simulink model "Ex1_Comparacion_con_SVC_Simulink"  (R2019a)
settings: Solver=VariableStepAuto  StartTime=0.0  StopTime=1  RelTol=1e-3
libraries: powerlib x53, powerlib_meascontrol x10, factslib x1
settings Model: Creator=USUARIO  LastModifiedBy=USUARIO

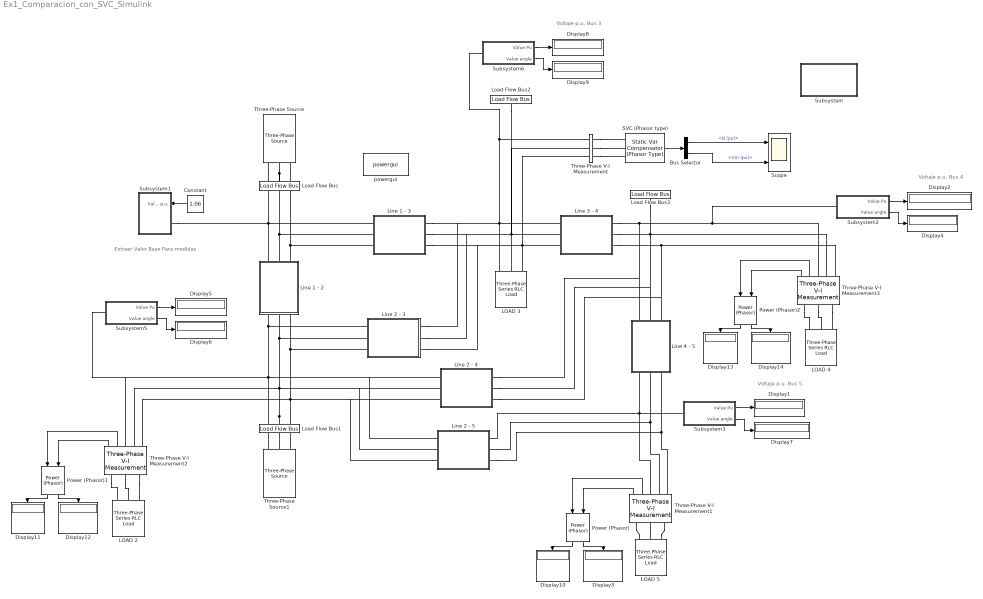
== system Ex1_Comparacion_con_SVC_Simulink ==
  note: Voltaje p.u. Bus 4
  note: Extraer Valor Base Para medidas
  note: Voltaje p.u. Bus 5
  note: Voltaje p.u. Bus 3
  Bus Selector : BusSelector  OutputSignals=Control.B (pu),Control.Vm (pu)
  Constant : Constant  Value=1.06
  Display{1..14} (14 alike) : Display
  LOAD 2 : powerlib/Elements/Three-Phase Series RLC Load  LConnTagsString=A|B|C  Configuration=Y (grounded)  NominalVoltage=(10000)*1  Vabc=[1e3 1e3 1e3]  Vabcp=[1e3 1e3 1e3]  NominalFrequency=60  UnbalancedPower=off  ActivePower=20e6  InductivePower=10e6  CapacitivePower=0  Pabc=[10e3 9e3 11e3]  QLabc=[100 90 110]  QCabc=[100 90 110]  Pabcp=[10e3 9e3 11e3]  QLabcp=[100 90 110]  QCabcp=[100 90 110]  Measurements=None  LoadType=constant PQ
      settings: SourceProductName=Simscape Electrical
  LOAD 3 : powerlib/Elements/Three-Phase Series RLC Load  LConnTagsString=A|B|C  Configuration=Y (grounded)  NominalVoltage=(10000)  Vabc=[1e3 1e3 1e3]  Vabcp=[1e3 1e3 1e3]  NominalFrequency=60  UnbalancedPower=off  ActivePower=45e6  InductivePower=15e6  CapacitivePower=0  Pabc=[10e3 9e3 11e3]  QLabc=[100 90 110]  QCabc=[100 90 110]  Pabcp=[10e3 9e3 11e3]  QLabcp=[100 90 110]  QCabcp=[100 90 110]  Measurements=None  LoadType=constant PQ
      settings: SourceProductName=Simscape Electrical
  LOAD 4 : powerlib/Elements/Three-Phase Series RLC Load  LConnTagsString=A|B|C  Configuration=Y (grounded)  NominalVoltage=(10000)*0.9943897  Vabc=[1e3 1e3 1e3]  Vabcp=[1e3 1e3 1e3]  NominalFrequency=60  UnbalancedPower=off  ActivePower=40e6  InductivePower=5e6  CapacitivePower=0  Pabc=[10e3 9e3 11e3]  QLabc=[100 90 110]  QCabc=[100 90 110]  Pabcp=[10e3 9e3 11e3]  QLabcp=[100 90 110]  QCabcp=[100 90 110]  Measurements=None  LoadType=constant PQ
      settings: SourceProductName=Simscape Electrical
  LOAD 5 : powerlib/Elements/Three-Phase Series RLC Load  LConnTagsString=A|B|C  Configuration=Y (grounded)  NominalVoltage=(10000)*0.9753  Vabc=[1e3 1e3 1e3]  Vabcp=[1e3 1e3 1e3]  NominalFrequency=60  UnbalancedPower=off  ActivePower=60e6  InductivePower=10e6  CapacitivePower=0  Pabc=[10e3 9e3 11e3]  QLabc=[100 90 110]  QCabc=[100 90 110]  Pabcp=[10e3 9e3 11e3]  QLabcp=[100 90 110]  QCabcp=[100 90 110]  Measurements=None  LoadType=constant PQ
      settings: SourceProductName=Simscape Electrical
  "Line 1 - 2 " : Subsystem  mask{F=60, R=0.02, XL=0.06, B=0.03}
      mask prompts: F "Frequency"; R "Resistance"; XL "Reactance"; B "Susceptance"
      mask Display: disp('Line')
  Line 1 - 3 : Subsystem  mask{F=60, R=0.08, XL=0.24, B=0.025}
      mask prompts: F "Frequency"; R "Resistance"; XL "Reactance"; B "Susceptance"
      mask Display: disp('Line')
  Line 2 - 3 : Subsystem  mask{F=60, R=0.06, XL=0.18, B=0.02}
      mask prompts: F "Frequency"; R "Resistance"; XL "Reactance"; B "Susceptance"
      mask Display: disp('Line')
  Line 2 - 4 : Subsystem  mask{F=60, R=0.06, XL=0.18, B=0.02}
      mask prompts: F "Frequency"; R "Resistance"; XL "Reactance"; B "Susceptance"
      mask Display: disp('Line')
  Line 2 - 5 : Subsystem  mask{F=60, R=0.04, XL=0.12, B=0.015}
      mask prompts: F "Frequency"; R "Resistance"; XL "Reactance"; B "Susceptance"
      mask Display: disp('Line')
  Line 3 - 4 : Subsystem  mask{F=60, R=0.01, XL=0.03, B=0.01}
      mask prompts: F "Frequency"; R "Resistance"; XL "Reactance"; B "Susceptance"
      mask Display: disp('Line')
  Line 4 - 5 : Subsystem  mask{F=60, R=0.08, XL=0.24, B=0.025}
      mask prompts: F "Frequency"; R "Resistance"; XL "Reactance"; B "Susceptance"
      mask Display: disp('Line')
  Load Flow Bus : powerlib/Measurements/Load Flow Bus  LConnTagsString=a  Phases=single  Connectors=on one side  ID=BUS_1  Vbase=10e3  Vref=1.06  Vangle=0  VLF=1.06  VLFb=1  VLFc=1  angleLF=0  angleLFb=0  angleLFc=0
      settings: SourceProductName=Simscape Electrical
  Load Flow Bus1 : powerlib/Measurements/Load Flow Bus  LConnTagsString=a  Phases=single  Connectors=on one side  ID=BUS_2  Vbase=10e3  Vref=1  Vangle=0  VLF=1  VLFb=1  VLFc=1  angleLF=-2.061  angleLFb=0  angleLFc=0
      settings: SourceProductName=Simscape Electrical
  Load Flow Bus2 : powerlib/Measurements/Load Flow Bus  LConnTagsString=a  Phases=single  Connectors=on one side  ID=BUS_3  Vbase=10e3  Vref=1  Vangle=0  VLF=0.9872  VLFb=1  VLFc=1  angleLF=-4.637  angleLFb=0  angleLFc=0
      settings: SourceProductName=Simscape Electrical
  Load Flow Bus3 : powerlib/Measurements/Load Flow Bus  LConnTagsString=a  Phases=single  Connectors=on one side  ID=BUS_4  Vbase=10e3  Vref=1  Vangle=0  VLF=0.9841  VLFb=1  VLFc=1  angleLF=-4.957  angleLFb=0  angleLFc=0
      settings: SourceProductName=Simscape Electrical
  Power (Phasor) : powerlib_meascontrol/Measurements/Power (Phasor)
      settings: SourceProductName=Simscape Electrical  SourceProductBaseCode=PS
  Power (Phasor)1 : powerlib_meascontrol/Measurements/Power (Phasor)
      settings: SourceProductName=Simscape Electrical  SourceProductBaseCode=PS
  Power (Phasor)2 : powerlib_meascontrol/Measurements/Power (Phasor)
      settings: SourceProductName=Simscape Electrical  SourceProductBaseCode=PS
  SVC (Phasor type) : factslib/Power-Electronics Based FACTS/Static Var Compensator (Phasor Type)  Seq1_Only=on  SystemNominal="[10e3  60]"  Pbase=200e6  Qnom="[200e6  -100e6]"  Td=4e-3  mode=Voltage regulation  Vref=1.0  ExternalVref=off  Xs=0  Kp_Ki=[0 300]  Bref=0.0
      settings: SourceProductName=Simscape Electrical  SourceProductBaseCode=PS
  Scope : Scope  NumInputPorts=2
  Subsystem : Subsystem
      mask Display: disp('Signal Processing')
  Subsystem1 : Subsystem
  Subsystem2 : Subsystem
  Subsystem3 : Subsystem
  Subsystem5 : Subsystem
  Subsystem6 : Subsystem
  Three-Phase V-I Measurement : powerlib/Measurements/Three-Phase V-I Measurement  VoltageMeasurement=phase-to-ground  SetLabelV=on  LabelV=Vabc  Vpu=on  VpuLL=off  CurrentMeasurement=yes  SetLabelI=on  LabelI=Iabc  Ipu=on  Pbase=100e6  Vbase=500e3  OutputType=Complex  PhasorSimulation=on  PSBequivalent=0
      settings: SourceProductName=Simscape Electrical
  Three-Phase V-I Measurement1 : powerlib/Measurements/Three-Phase V-I Measurement  VoltageMeasurement=phase-to-ground  SetLabelV=off  LabelV=Vabc  Vpu=off  VpuLL=off  CurrentMeasurement=yes  SetLabelI=off  LabelI=Iabc  Ipu=off  Pbase=100e6  Vbase=500e3  OutputType=Complex  PhasorSimulation=on  PSBequivalent=0
      settings: SourceProductName=Simscape Electrical
  Three-Phase V-I Measurement2 : powerlib/Measurements/Three-Phase V-I Measurement  VoltageMeasurement=phase-to-ground  SetLabelV=off  LabelV=Vabc  Vpu=off  VpuLL=off  CurrentMeasurement=yes  SetLabelI=off  LabelI=Iabc  Ipu=off  Pbase=100e6  Vbase=500e3  OutputType=Complex  PhasorSimulation=on  PSBequivalent=0
      settings: SourceProductName=Simscape Electrical
  Three-Phase V-I Measurement3 : powerlib/Measurements/Three-Phase V-I Measurement  VoltageMeasurement=phase-to-ground  SetLabelV=off  LabelV=Vabc  Vpu=off  VpuLL=off  CurrentMeasurement=yes  SetLabelI=off  LabelI=Iabc  Ipu=off  Pbase=100e6  Vbase=500e3  OutputType=Complex  PhasorSimulation=on  PSBequivalent=0
      settings: SourceProductName=Simscape Electrical
  Three-Phase Source : powerlib/Electrical Sources/Three-Phase Source  InternalConnection=Yg  VoltagePhases=off  Voltage=(10000)*1.06  PhaseAngle=0  Voltage_phases=[25e3 25e3 25e3]/sqrt(3)  PhaseAngles_phases=[0 -120 +120]  Frequency=60  NonIdealSource=off  SpecifyImpedance=off  Resistance=1e-5  Inductance=0  ShortCircuitLevel=100e6  BaseVoltage=10e3  XRratio=7  BusType=swing  Pref=10e3  Qref=0  Prefabc=[10e3, 10e3, 10e3]  Qrefabc=[0, 0, 0]  Qmin=-inf  Qmax=inf
      settings: SourceProductName=Simscape Electrical
  Three-Phase Source1 : powerlib/Electrical Sources/Three-Phase Source  InternalConnection=Yg  VoltagePhases=off  Voltage=(10000)*1  PhaseAngle=-2.053  Voltage_phases=[25e3 25e3 25e3]/sqrt(3)  PhaseAngles_phases=[0 -120 +120]  Frequency=60  NonIdealSource=off  SpecifyImpedance=off  Resistance=0.8929  Inductance=16.58e-3  ShortCircuitLevel=100e6  BaseVoltage=25e3  XRratio=7  BusType=PV  Pref=40e6  Qref=0  Prefabc=[10e3, 10e3, 10e3]  Qrefabc=[0, 0, 0]  Qmin=-inf  Qmax=inf
      settings: SourceProductName=Simscape Electrical
  powergui : powerlib/powergui  Priority=1  SimulationMode=Phasor  SampleTime=50e-6  frequency=60  Iterations=50  frequencyindice=60  Pbase=100e6  ErrMax=1e-12  UnitsV=kV  UnitsW=MW  buscounter=0  FunctionMessages=off  echomessages=off  EnableUseOfTLC=off  CurrentSourceSwitches=off  DisableSnubberDevices=off  DisableRonSwitches=off  DisableVfSwitches=off  DisplayEquations=off  AutomaticDiscreteSolvers=off  SolverType=Tustin/Backward Euler (TBE)  Interpol=off  ExternalGateDelay=off  methode=off  Ts=100  x0status=blocks  SPID=on  SwTol=0  HookPort=off  NonlinearTolerance=0  nMaxIteration=15  ContinueOnMaxIteration=off  RestoreLinks=warning  ResistiveCurrentMeasurement=off  Frange=[0:2:500]  Ylog=off  Xlog=on  ShowGrid=off  save=off  variable=ZData  structure=0  ZoomFFT=off  StartTime=0.0  cycles=1  DisplayStyle=1  fundamental=60  FreqAxis=off  MaxFrequency=1000  frequencyindicesteady=1  RmsSteady=1  display=off
      settings: SourceProductName=Simscape Electrical
  wires:
  SVC (Phasor type)/1 -> Bus Selector/1
  Bus Selector/2 -> Scope/2  "<Vm (pu)>"
  Bus Selector/1 -> Scope/1  "<B (pu)>"
  Constant/1 -> Subsystem1/1(Value p.u.)
  Subsystem2/2(Value angle) -> Display4/1
  Subsystem5/2(Value angle) -> Display6/1
  Subsystem5/1("Value Pu ") -> Display5/1
  Subsystem3/2(Value angle) -> Display7/1
  Subsystem3/1("Value Pu ") -> Display1/1
  Subsystem6/1("Value Pu ") -> Display8/1
  Subsystem6/2(Value angle) -> Display9/1
  Subsystem2/1("Value Pu ") -> Display2/1
  Power (Phasor)/2 -> Display10/1
  Power (Phasor)/1 -> Display3/1
  Three-Phase V-I Measurement1/1 -> Power (Phasor)/1
  Three-Phase V-I Measurement1/2 -> Power (Phasor)/2
  Three-Phase V-I Measurement2/2 -> Power (Phasor)1/2
  Power (Phasor)1/1 -> Display12/1
  Power (Phasor)1/2 -> Display11/1
  Three-Phase V-I Measurement2/1 -> Power (Phasor)1/1
  Three-Phase V-I Measurement3/2 -> Power (Phasor)2/2
  Power (Phasor)2/1 -> Display14/1
  Power (Phasor)2/2 -> Display13/1
  Three-Phase V-I Measurement3/1 -> Power (Phasor)2/1
  connections:
  Three-Phase Source1/RConn1 -- Three-Phase V-I Measurement2/RConn1 -- Subsystem5/LConn1 -- Line 2 - 5/LConn1 -- Line 2 - 4/LConn1 -- "Line 1 - 2 "/RConn1 -- Line 2 - 3/LConn1
  Three-Phase Source1/RConn2 -- Load Flow Bus1/LConn1 -- Three-Phase V-I Measurement2/RConn2 -- Line 2 - 4/LConn2 -- Line 2 - 5/LConn2 -- "Line 1 - 2 "/RConn2 -- Line 2 - 3/LConn2
  Three-Phase Source1/RConn3 -- Three-Phase V-I Measurement2/RConn3 -- "Line 1 - 2 "/RConn3 -- Line 2 - 3/LConn3 -- Line 2 - 4/LConn3 -- Line 2 - 5/LConn3
  Load Flow Bus/LConn1 -- Line 1 - 3/LConn2 -- "Line 1 - 2 "/LConn2 -- Three-Phase Source/RConn2
  Line 1 - 3/LConn3 -- Three-Phase Source/RConn3 -- "Line 1 - 2 "/LConn3
  LOAD 3/LConn1 -- Subsystem6/LConn1 -- Three-Phase V-I Measurement/LConn1 -- Line 3 - 4/LConn1 -- Line 2 - 3/RConn1 -- Line 1 - 3/RConn1
  LOAD 3/LConn2 -- Load Flow Bus2/LConn1 -- Three-Phase V-I Measurement/LConn2 -- Line 3 - 4/LConn2 -- Line 2 - 3/RConn2 -- Line 1 - 3/RConn2
  LOAD 3/LConn3 -- Three-Phase V-I Measurement/LConn3 -- Line 3 - 4/LConn3 -- Line 2 - 3/RConn3 -- Line 1 - 3/RConn3
  Line 3 - 4/RConn1 -- Line 4 - 5/LConn1 -- Line 2 - 4/RConn1 -- Three-Phase V-I Measurement3/RConn1 -- Subsystem2/LConn1
  Line 3 - 4/RConn2 -- Three-Phase V-I Measurement3/RConn2 -- Load Flow Bus3/LConn1 -- Line 4 - 5/LConn2 -- Line 2 - 4/RConn2
  Line 3 - 4/RConn3 -- Three-Phase V-I Measurement3/RConn3 -- Line 2 - 4/RConn3 -- Line 4 - 5/LConn3
  Line 2 - 5/RConn1 -- Three-Phase V-I Measurement1/RConn1 -- Subsystem3/LConn1 -- Line 4 - 5/RConn1
  Line 2 - 5/RConn2 -- Three-Phase V-I Measurement1/RConn2 -- Line 4 - 5/RConn2
  Line 2 - 5/RConn3 -- Three-Phase V-I Measurement1/RConn3 -- Line 4 - 5/RConn3
  Three-Phase V-I Measurement/RConn2 -- SVC (Phasor type)/LConn2
  Three-Phase V-I Measurement/RConn3 -- SVC (Phasor type)/LConn3
  Three-Phase V-I Measurement/RConn1 -- SVC (Phasor type)/LConn1
  Line 1 - 3/LConn1 -- Subsystem1/LConn1 -- Three-Phase Source/RConn1 -- "Line 1 - 2 "/LConn1
  Three-Phase V-I Measurement1/LConn1 -- LOAD 5/LConn1
  Three-Phase V-I Measurement1/LConn2 -- LOAD 5/LConn2
  Three-Phase V-I Measurement1/LConn3 -- LOAD 5/LConn3
  Three-Phase V-I Measurement2/LConn3 -- LOAD 2/LConn3
  Three-Phase V-I Measurement2/LConn1 -- LOAD 2/LConn1
  Three-Phase V-I Measurement2/LConn2 -- LOAD 2/LConn2
  Three-Phase V-I Measurement3/LConn1 -- LOAD 4/LConn1
  Three-Phase V-I Measurement3/LConn2 -- LOAD 4/LConn2
  Three-Phase V-I Measurement3/LConn3 -- LOAD 4/LConn3

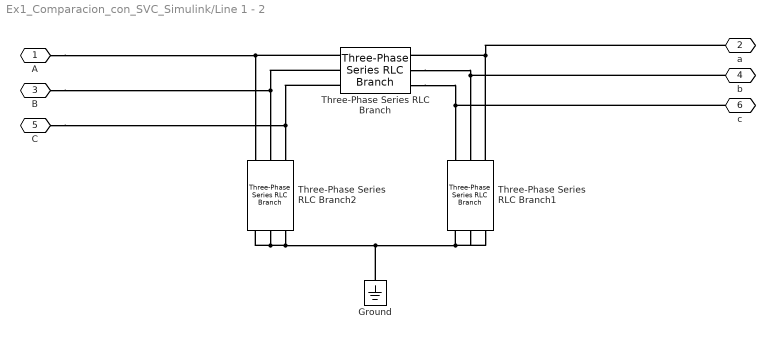
== system Ex1_Comparacion_con_SVC_Simulink/Line 1 - 2  ==
  Ground : powerlib/Elements/Ground  LConnTagsString=a
      settings: SourceProductName=Simscape Electrical
  Three-Phase Series RLC Branch : powerlib/Elements/Three-Phase Series RLC Branch  LConnTagsString=A|B|C  RConnTagsString=A|B|C  BranchType=RL  Resistance=R  Inductance=XL/(2*pi*F)  Capacitance=0  Measurements=None
      settings: SourceProductName=Simscape Electrical
  Three-Phase Series RLC Branch1 : powerlib/Elements/Three-Phase Series RLC Branch  LConnTagsString=A|B|C  RConnTagsString=A|B|C  BranchType=RC  Resistance=1e-5  Inductance=0  Capacitance=B/(2*pi*F)  Measurements=None
      settings: SourceProductName=Simscape Electrical
  Three-Phase Series RLC Branch2 : powerlib/Elements/Three-Phase Series RLC Branch  LConnTagsString=A|B|C  RConnTagsString=A|B|C  BranchType=RC  Resistance=1e-5  Inductance=0  Capacitance=B/(2*pi*F)  Measurements=None
      settings: SourceProductName=Simscape Electrical
  A : PMIOPort  Side=Left
  a : PMIOPort  Port=2  Side=Right
  B : PMIOPort  Port=3  Side=Left
  b : PMIOPort  Port=4  Side=Right
  C : PMIOPort  Port=5  Side=Left
  c : PMIOPort  Port=6  Side=Right
  connections:
  Three-Phase Series RLC Branch/RConn3 -- c/RConn1 -- Three-Phase Series RLC Branch1/LConn1
  Three-Phase Series RLC Branch2/RConn3 -- Ground/LConn1 -- Three-Phase Series RLC Branch1/RConn3 -- Three-Phase Series RLC Branch1/RConn2 -- Three-Phase Series RLC Branch1/RConn1 -- Three-Phase Series RLC Branch2/RConn2 -- Three-Phase Series RLC Branch2/RConn1
  Three-Phase Series RLC Branch/LConn3 -- C/RConn1 -- Three-Phase Series RLC Branch2/LConn3
  Three-Phase Series RLC Branch1/LConn3 -- a/RConn1 -- Three-Phase Series RLC Branch/RConn1
  Three-Phase Series RLC Branch/RConn2 -- b/RConn1 -- Three-Phase Series RLC Branch1/LConn2
  Three-Phase Series RLC Branch/LConn2 -- B/RConn1 -- Three-Phase Series RLC Branch2/LConn2
  Three-Phase Series RLC Branch/LConn1 -- A/RConn1 -- Three-Phase Series RLC Branch2/LConn1

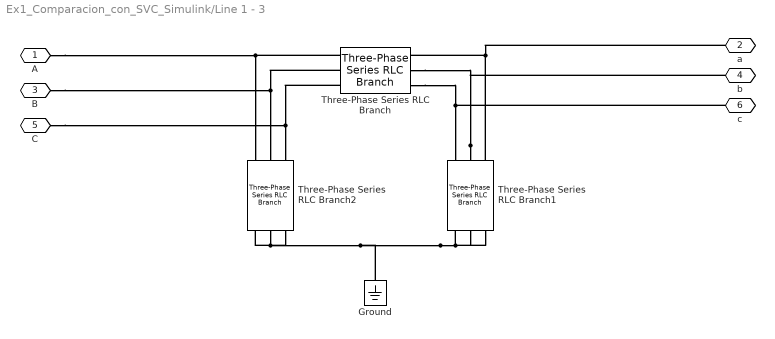
== system Ex1_Comparacion_con_SVC_Simulink/Line 1 - 3 ==
  Ground : powerlib/Elements/Ground  LConnTagsString=a
      settings: SourceProductName=Simscape Electrical
  Three-Phase Series RLC Branch : powerlib/Elements/Three-Phase Series RLC Branch  LConnTagsString=A|B|C  RConnTagsString=A|B|C  BranchType=RL  Resistance=R  Inductance=XL/(2*pi*F)  Capacitance=0  Measurements=None
      settings: SourceProductName=Simscape Electrical
  Three-Phase Series RLC Branch1 : powerlib/Elements/Three-Phase Series RLC Branch  LConnTagsString=A|B|C  RConnTagsString=A|B|C  BranchType=C  Resistance=0  Inductance=0  Capacitance=B/(2*pi*F)  Measurements=None
      settings: SourceProductName=Simscape Electrical
  Three-Phase Series RLC Branch2 : powerlib/Elements/Three-Phase Series RLC Branch  LConnTagsString=A|B|C  RConnTagsString=A|B|C  BranchType=RC  Resistance=1e-5  Inductance=0  Capacitance=B/(2*pi*F)  Measurements=None
      settings: SourceProductName=Simscape Electrical
  A : PMIOPort  Side=Left
  a : PMIOPort  Port=2  Side=Right
  B : PMIOPort  Port=3  Side=Left
  b : PMIOPort  Port=4  Side=Right
  C : PMIOPort  Port=5  Side=Left
  c : PMIOPort  Port=6  Side=Right
  connections:
  Three-Phase Series RLC Branch/RConn3 -- Three-Phase Series RLC Branch1/LConn1 -- c/RConn1
  Three-Phase Series RLC Branch2/RConn2 -- Three-Phase Series RLC Branch2/RConn1 -- Three-Phase Series RLC Branch2/RConn3 -- Three-Phase Series RLC Branch1/RConn3 -- Three-Phase Series RLC Branch1/RConn2 -- Three-Phase Series RLC Branch1/RConn1 -- Ground/LConn1
  Three-Phase Series RLC Branch/LConn3 -- Three-Phase Series RLC Branch2/LConn3 -- C/RConn1
  Three-Phase Series RLC Branch1/LConn3 -- Three-Phase Series RLC Branch/RConn1 -- a/RConn1
  Three-Phase Series RLC Branch1/LConn2 -- Three-Phase Series RLC Branch/RConn2 -- b/RConn1
  Three-Phase Series RLC Branch/LConn2 -- Three-Phase Series RLC Branch2/LConn2 -- B/RConn1
  Three-Phase Series RLC Branch/LConn1 -- Three-Phase Series RLC Branch2/LConn1 -- A/RConn1

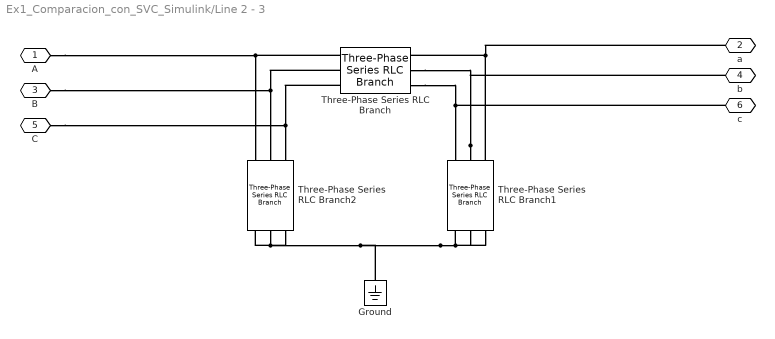
== system Ex1_Comparacion_con_SVC_Simulink/Line 2 - 3 ==
  Ground : powerlib/Elements/Ground  LConnTagsString=a
      settings: SourceProductName=Simscape Electrical
  Three-Phase Series RLC Branch : powerlib/Elements/Three-Phase Series RLC Branch  LConnTagsString=A|B|C  RConnTagsString=A|B|C  BranchType=RL  Resistance=R  Inductance=XL/(2*pi*F)  Capacitance=0  Measurements=None
      settings: SourceProductName=Simscape Electrical
  Three-Phase Series RLC Branch1 : powerlib/Elements/Three-Phase Series RLC Branch  LConnTagsString=A|B|C  RConnTagsString=A|B|C  BranchType=C  Resistance=0  Inductance=0  Capacitance=B/(2*pi*F)  Measurements=None
      settings: SourceProductName=Simscape Electrical
  Three-Phase Series RLC Branch2 : powerlib/Elements/Three-Phase Series RLC Branch  LConnTagsString=A|B|C  RConnTagsString=A|B|C  BranchType=RC  Resistance=1e-5  Inductance=0  Capacitance=B/(2*pi*F)  Measurements=None
      settings: SourceProductName=Simscape Electrical
  A : PMIOPort  Side=Left
  a : PMIOPort  Port=2  Side=Right
  B : PMIOPort  Port=3  Side=Left
  b : PMIOPort  Port=4  Side=Right
  C : PMIOPort  Port=5  Side=Left
  c : PMIOPort  Port=6  Side=Right
  connections:
  Three-Phase Series RLC Branch/RConn3 -- Three-Phase Series RLC Branch1/LConn1 -- c/RConn1
  Three-Phase Series RLC Branch2/RConn2 -- Three-Phase Series RLC Branch2/RConn1 -- Three-Phase Series RLC Branch2/RConn3 -- Three-Phase Series RLC Branch1/RConn3 -- Three-Phase Series RLC Branch1/RConn2 -- Three-Phase Series RLC Branch1/RConn1 -- Ground/LConn1
  Three-Phase Series RLC Branch/LConn3 -- Three-Phase Series RLC Branch2/LConn3 -- C/RConn1
  Three-Phase Series RLC Branch1/LConn3 -- Three-Phase Series RLC Branch/RConn1 -- a/RConn1
  Three-Phase Series RLC Branch1/LConn2 -- Three-Phase Series RLC Branch/RConn2 -- b/RConn1
  Three-Phase Series RLC Branch/LConn2 -- Three-Phase Series RLC Branch2/LConn2 -- B/RConn1
  Three-Phase Series RLC Branch/LConn1 -- Three-Phase Series RLC Branch2/LConn1 -- A/RConn1

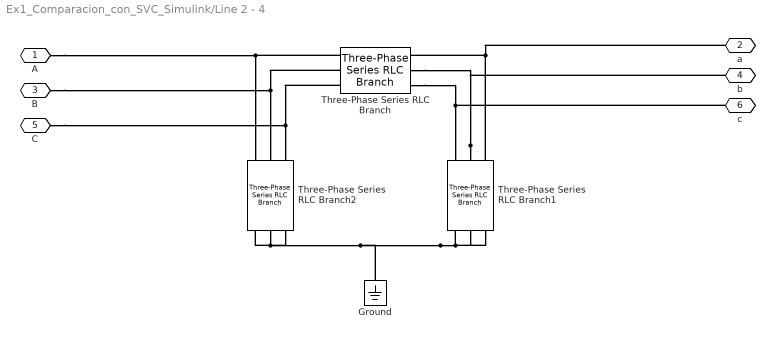
== system Ex1_Comparacion_con_SVC_Simulink/Line 2 - 4 ==
  Ground : powerlib/Elements/Ground  LConnTagsString=a
      settings: SourceProductName=Simscape Electrical
  Three-Phase Series RLC Branch : powerlib/Elements/Three-Phase Series RLC Branch  LConnTagsString=A|B|C  RConnTagsString=A|B|C  BranchType=RL  Resistance=R  Inductance=XL/(2*pi*F)  Capacitance=0  Measurements=None
      settings: SourceProductName=Simscape Electrical
  Three-Phase Series RLC Branch1 : powerlib/Elements/Three-Phase Series RLC Branch  LConnTagsString=A|B|C  RConnTagsString=A|B|C  BranchType=C  Resistance=0  Inductance=0  Capacitance=B/(2*pi*F)  Measurements=None
      settings: SourceProductName=Simscape Electrical
  Three-Phase Series RLC Branch2 : powerlib/Elements/Three-Phase Series RLC Branch  LConnTagsString=A|B|C  RConnTagsString=A|B|C  BranchType=RC  Resistance=1e-5  Inductance=0  Capacitance=B/(2*pi*F)  Measurements=None
      settings: SourceProductName=Simscape Electrical
  A : PMIOPort  Side=Left
  a : PMIOPort  Port=2  Side=Right
  B : PMIOPort  Port=3  Side=Left
  b : PMIOPort  Port=4  Side=Right
  C : PMIOPort  Port=5  Side=Left
  c : PMIOPort  Port=6  Side=Right
  connections:
  Three-Phase Series RLC Branch/RConn3 -- Three-Phase Series RLC Branch1/LConn1 -- c/RConn1
  Three-Phase Series RLC Branch2/RConn2 -- Three-Phase Series RLC Branch2/RConn1 -- Three-Phase Series RLC Branch2/RConn3 -- Three-Phase Series RLC Branch1/RConn3 -- Three-Phase Series RLC Branch1/RConn2 -- Three-Phase Series RLC Branch1/RConn1 -- Ground/LConn1
  Three-Phase Series RLC Branch/LConn3 -- Three-Phase Series RLC Branch2/LConn3 -- C/RConn1
  Three-Phase Series RLC Branch1/LConn3 -- Three-Phase Series RLC Branch/RConn1 -- a/RConn1
  Three-Phase Series RLC Branch1/LConn2 -- Three-Phase Series RLC Branch/RConn2 -- b/RConn1
  Three-Phase Series RLC Branch/LConn2 -- Three-Phase Series RLC Branch2/LConn2 -- B/RConn1
  Three-Phase Series RLC Branch/LConn1 -- Three-Phase Series RLC Branch2/LConn1 -- A/RConn1

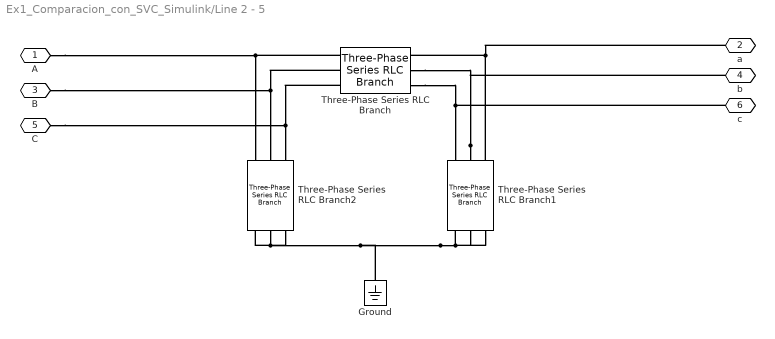
== system Ex1_Comparacion_con_SVC_Simulink/Line 2 - 5 ==
  Ground : powerlib/Elements/Ground  LConnTagsString=a
      settings: SourceProductName=Simscape Electrical
  Three-Phase Series RLC Branch : powerlib/Elements/Three-Phase Series RLC Branch  LConnTagsString=A|B|C  RConnTagsString=A|B|C  BranchType=RL  Resistance=R  Inductance=XL/(2*pi*F)  Capacitance=0  Measurements=None
      settings: SourceProductName=Simscape Electrical
  Three-Phase Series RLC Branch1 : powerlib/Elements/Three-Phase Series RLC Branch  LConnTagsString=A|B|C  RConnTagsString=A|B|C  BranchType=C  Resistance=0  Inductance=0  Capacitance=B/(2*pi*F)  Measurements=None
      settings: SourceProductName=Simscape Electrical
  Three-Phase Series RLC Branch2 : powerlib/Elements/Three-Phase Series RLC Branch  LConnTagsString=A|B|C  RConnTagsString=A|B|C  BranchType=RC  Resistance=1e-5  Inductance=0  Capacitance=B/(2*pi*F)  Measurements=None
      settings: SourceProductName=Simscape Electrical
  A : PMIOPort  Side=Left
  a : PMIOPort  Port=2  Side=Right
  B : PMIOPort  Port=3  Side=Left
  b : PMIOPort  Port=4  Side=Right
  C : PMIOPort  Port=5  Side=Left
  c : PMIOPort  Port=6  Side=Right
  connections:
  Three-Phase Series RLC Branch/RConn3 -- Three-Phase Series RLC Branch1/LConn1 -- c/RConn1
  Three-Phase Series RLC Branch2/RConn2 -- Three-Phase Series RLC Branch2/RConn1 -- Three-Phase Series RLC Branch2/RConn3 -- Three-Phase Series RLC Branch1/RConn3 -- Three-Phase Series RLC Branch1/RConn2 -- Three-Phase Series RLC Branch1/RConn1 -- Ground/LConn1
  Three-Phase Series RLC Branch/LConn3 -- Three-Phase Series RLC Branch2/LConn3 -- C/RConn1
  Three-Phase Series RLC Branch1/LConn3 -- Three-Phase Series RLC Branch/RConn1 -- a/RConn1
  Three-Phase Series RLC Branch1/LConn2 -- Three-Phase Series RLC Branch/RConn2 -- b/RConn1
  Three-Phase Series RLC Branch/LConn2 -- Three-Phase Series RLC Branch2/LConn2 -- B/RConn1
  Three-Phase Series RLC Branch/LConn1 -- Three-Phase Series RLC Branch2/LConn1 -- A/RConn1

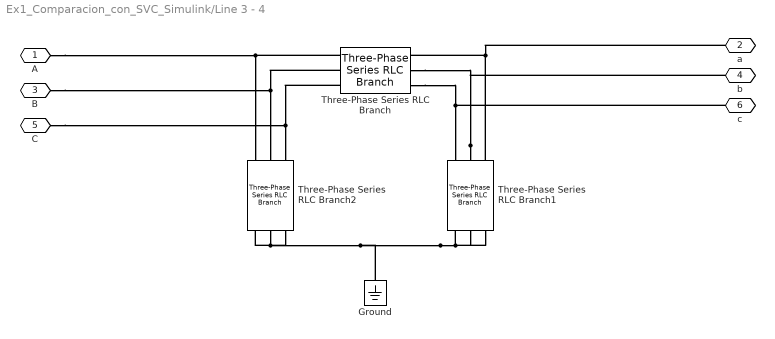
== system Ex1_Comparacion_con_SVC_Simulink/Line 3 - 4 ==
  Ground : powerlib/Elements/Ground  LConnTagsString=a
      settings: SourceProductName=Simscape Electrical
  Three-Phase Series RLC Branch : powerlib/Elements/Three-Phase Series RLC Branch  LConnTagsString=A|B|C  RConnTagsString=A|B|C  BranchType=RL  Resistance=R  Inductance=XL/(2*pi*F)  Capacitance=0  Measurements=None
      settings: SourceProductName=Simscape Electrical
  Three-Phase Series RLC Branch1 : powerlib/Elements/Three-Phase Series RLC Branch  LConnTagsString=A|B|C  RConnTagsString=A|B|C  BranchType=C  Resistance=0  Inductance=0  Capacitance=B/(2*pi*F)  Measurements=None
      settings: SourceProductName=Simscape Electrical
  Three-Phase Series RLC Branch2 : powerlib/Elements/Three-Phase Series RLC Branch  LConnTagsString=A|B|C  RConnTagsString=A|B|C  BranchType=C  Resistance=0  Inductance=0  Capacitance=B/(2*pi*F)  Measurements=None
      settings: SourceProductName=Simscape Electrical
  A : PMIOPort  Side=Left
  a : PMIOPort  Port=2  Side=Right
  B : PMIOPort  Port=3  Side=Left
  b : PMIOPort  Port=4  Side=Right
  C : PMIOPort  Port=5  Side=Left
  c : PMIOPort  Port=6  Side=Right
  connections:
  Three-Phase Series RLC Branch/RConn3 -- Three-Phase Series RLC Branch1/LConn1 -- c/RConn1
  Three-Phase Series RLC Branch2/RConn2 -- Three-Phase Series RLC Branch2/RConn1 -- Three-Phase Series RLC Branch2/RConn3 -- Three-Phase Series RLC Branch1/RConn3 -- Three-Phase Series RLC Branch1/RConn2 -- Three-Phase Series RLC Branch1/RConn1 -- Ground/LConn1
  Three-Phase Series RLC Branch/LConn3 -- Three-Phase Series RLC Branch2/LConn3 -- C/RConn1
  Three-Phase Series RLC Branch1/LConn3 -- Three-Phase Series RLC Branch/RConn1 -- a/RConn1
  Three-Phase Series RLC Branch1/LConn2 -- Three-Phase Series RLC Branch/RConn2 -- b/RConn1
  Three-Phase Series RLC Branch/LConn2 -- Three-Phase Series RLC Branch2/LConn2 -- B/RConn1
  Three-Phase Series RLC Branch/LConn1 -- Three-Phase Series RLC Branch2/LConn1 -- A/RConn1

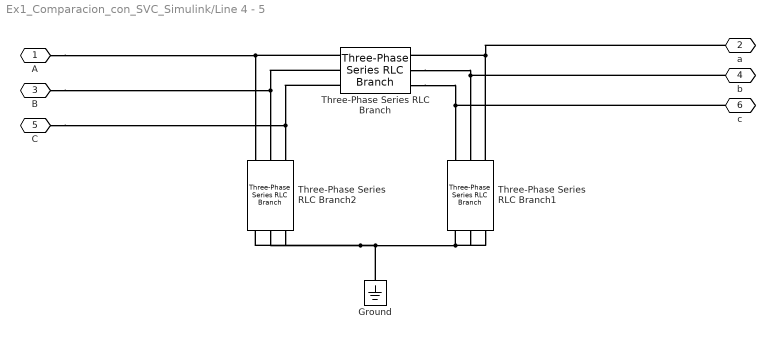
== system Ex1_Comparacion_con_SVC_Simulink/Line 4 - 5 ==
  Ground : powerlib/Elements/Ground  LConnTagsString=a
      settings: SourceProductName=Simscape Electrical
  Three-Phase Series RLC Branch : powerlib/Elements/Three-Phase Series RLC Branch  LConnTagsString=A|B|C  RConnTagsString=A|B|C  BranchType=RL  Resistance=R  Inductance=XL/(2*pi*F)  Capacitance=0  Measurements=None
      settings: SourceProductName=Simscape Electrical
  Three-Phase Series RLC Branch1 : powerlib/Elements/Three-Phase Series RLC Branch  LConnTagsString=A|B|C  RConnTagsString=A|B|C  BranchType=C  Resistance=0  Inductance=0  Capacitance=B/(2*pi*F)  Measurements=None
      settings: SourceProductName=Simscape Electrical
  Three-Phase Series RLC Branch2 : powerlib/Elements/Three-Phase Series RLC Branch  LConnTagsString=A|B|C  RConnTagsString=A|B|C  BranchType=C  Resistance=0  Inductance=0  Capacitance=B/(2*pi*F)  Measurements=None
      settings: SourceProductName=Simscape Electrical
  A : PMIOPort  Side=Left
  a : PMIOPort  Port=2  Side=Right
  B : PMIOPort  Port=3  Side=Left
  b : PMIOPort  Port=4  Side=Right
  C : PMIOPort  Port=5  Side=Left
  c : PMIOPort  Port=6  Side=Right
  connections:
  A/RConn1 -- Three-Phase Series RLC Branch2/LConn1 -- Three-Phase Series RLC Branch/LConn1
  B/RConn1 -- Three-Phase Series RLC Branch2/LConn2 -- Three-Phase Series RLC Branch/LConn2
  b/RConn1 -- Three-Phase Series RLC Branch/RConn2 -- Three-Phase Series RLC Branch1/LConn2
  a/RConn1 -- Three-Phase Series RLC Branch/RConn1 -- Three-Phase Series RLC Branch1/LConn3
  C/RConn1 -- Three-Phase Series RLC Branch2/LConn3 -- Three-Phase Series RLC Branch/LConn3
  Ground/LConn1 -- Three-Phase Series RLC Branch1/RConn1 -- Three-Phase Series RLC Branch1/RConn2 -- Three-Phase Series RLC Branch1/RConn3 -- Three-Phase Series RLC Branch2/RConn3 -- Three-Phase Series RLC Branch2/RConn1 -- Three-Phase Series RLC Branch2/RConn2
  c/RConn1 -- Three-Phase Series RLC Branch1/LConn1 -- Three-Phase Series RLC Branch/RConn3

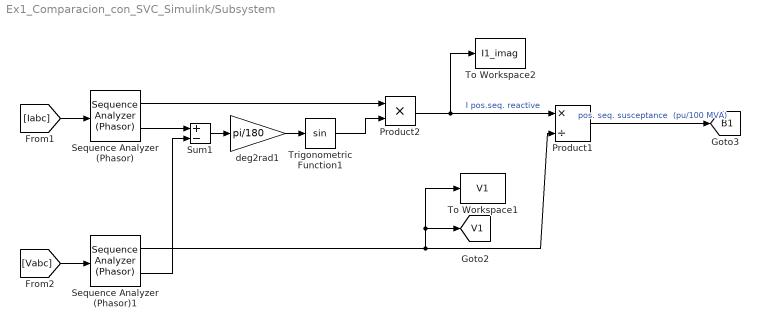
== system Ex1_Comparacion_con_SVC_Simulink/Subsystem ==
  Product1 : Product  Inputs=*/  SaturateOnIntegerOverflow=on  OutDataTypeStr=Inherit: Same as first input
  Product2 : Product  Inputs=**  SaturateOnIntegerOverflow=on  OutDataTypeStr=Inherit: Same as first input
  Sequence Analyzer (Phasor) : powerlib_meascontrol/Measurements/Sequence Analyzer (Phasor)  seq=Positive
      settings: SourceProductName=Simscape Electrical  SourceProductBaseCode=PS
  Sequence Analyzer (Phasor)1 : powerlib_meascontrol/Measurements/Sequence Analyzer (Phasor)  seq=Positive
      settings: SourceProductName=Simscape Electrical  SourceProductBaseCode=PS
  Sum1 : Sum  Inputs=+-  SaturateOnIntegerOverflow=on
  To Workspace1 : ToWorkspace  VariableName=V1  SampleTime=-1
  To Workspace2 : ToWorkspace  VariableName=I1_imag  SampleTime=-1
  Trigonometric Function1 : Trigonometry
  deg2rad1 : Gain  Gain=pi/180  SaturateOnIntegerOverflow=on  OutDataTypeStr=Inherit: Same as input  ParamDataTypeStr=Inherit: Same as input
  tag scope: B1=global, V1=global
  wires:
  Sequence Analyzer (Phasor)1/1 -> Product1/2, To Workspace1/1, [V1]
  Product1/1 -> [B1]  "pos. seq. susceptance  (pu/100 MVA)"
  [Iabc] -> Sequence Analyzer (Phasor)/1
  [Vabc] -> Sequence Analyzer (Phasor)1/1
  Sum1/1 -> deg2rad1/1
  deg2rad1/1 -> Trigonometric Function1/1
  Sequence Analyzer (Phasor)1/2 -> Sum1/2
  Sequence Analyzer (Phasor)/2 -> Sum1/1
  Trigonometric Function1/1 -> Product2/2
  Product2/1 -> Product1/1, To Workspace2/1  "I pos.seq. reactive"
  Sequence Analyzer (Phasor)/1 -> Product2/1

== system Ex1_Comparacion_con_SVC_Simulink/Subsystem1 ==
  Value p.u. : Inport
  Display1 : Display
  Divide : Product  Inputs=*/
  Ground1 : powerlib/Elements/Ground  LConnTagsString=a
      settings: SourceProductName=Simscape Electrical
  RMS1 : powerlib_meascontrol/Measurements/RMS  TrueRMS=on  Freq=60  RMSInit=120  Ts=0
      settings: SourceProductName=Simscape Electrical
  Voltage Measurement1 : powerlib/Measurements/Voltage Measurement  PhasorSimulation=on  OutputType=Magnitude  PSBequivalent=0
      settings: SourceProductName=Simscape Electrical
  VMeasure : PMIOPort  Side=Left
  tag scope: VbaseRMS=global
  wires:
  Voltage Measurement1/1 -> RMS1/1
  Divide/1 -> [VbaseRMS]
  RMS1/1 -> Divide/1, Display1/1
  Value p.u./1 -> Divide/2
  connections:
  Voltage Measurement1/LConn1 -- VMeasure/RConn1
  Ground1/LConn1 -- Voltage Measurement1/LConn2

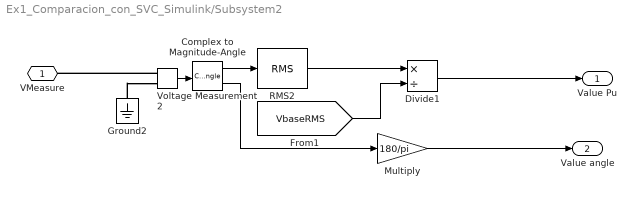
== system Ex1_Comparacion_con_SVC_Simulink/Subsystem2 ==
  Complex to Magnitude-Angle : ComplexToMagnitudeAngle
  Divide1 : Product  Inputs=*/
  Ground2 : powerlib/Elements/Ground  LConnTagsString=a
      settings: SourceProductName=Simscape Electrical
  Multiply : Gain  Gain=180/pi
  RMS2 : powerlib_meascontrol/Measurements/RMS  TrueRMS=on  Freq=60  RMSInit=120  Ts=0
      settings: SourceProductName=Simscape Electrical
  Voltage Measurement2 : powerlib/Measurements/Voltage Measurement  PhasorSimulation=on  OutputType=Complex  PSBequivalent=0
      settings: SourceProductName=Simscape Electrical
  VMeasure : PMIOPort  Side=Left
  "Value Pu " : Outport
  Value angle : Outport  Port=2
  wires:
  RMS2/1 -> Divide1/1
  Divide1/1 -> "Value Pu "/1
  [VbaseRMS] -> Divide1/2
  Voltage Measurement2/1 -> Complex to Magnitude-Angle/1
  Complex to Magnitude-Angle/1 -> RMS2/1
  Multiply/1 -> Value angle/1
  Complex to Magnitude-Angle/2 -> Multiply/1
  connections:
  Ground2/LConn1 -- Voltage Measurement2/LConn2
  Voltage Measurement2/LConn1 -- VMeasure/RConn1

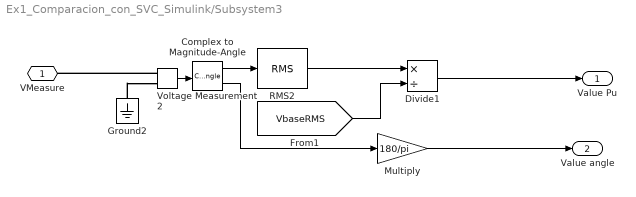
== system Ex1_Comparacion_con_SVC_Simulink/Subsystem3 ==
  Complex to Magnitude-Angle : ComplexToMagnitudeAngle
  Divide1 : Product  Inputs=*/
  Ground2 : powerlib/Elements/Ground  LConnTagsString=a
      settings: SourceProductName=Simscape Electrical
  Multiply : Gain  Gain=180/pi
  RMS2 : powerlib_meascontrol/Measurements/RMS  TrueRMS=on  Freq=60  RMSInit=120  Ts=0
      settings: SourceProductName=Simscape Electrical
  Voltage Measurement2 : powerlib/Measurements/Voltage Measurement  PhasorSimulation=on  OutputType=Complex  PSBequivalent=0
      settings: SourceProductName=Simscape Electrical
  VMeasure : PMIOPort  Side=Left
  "Value Pu " : Outport
  Value angle : Outport  Port=2
  wires:
  RMS2/1 -> Divide1/1
  Divide1/1 -> "Value Pu "/1
  [VbaseRMS] -> Divide1/2
  Voltage Measurement2/1 -> Complex to Magnitude-Angle/1
  Complex to Magnitude-Angle/1 -> RMS2/1
  Multiply/1 -> Value angle/1
  Complex to Magnitude-Angle/2 -> Multiply/1
  connections:
  Ground2/LConn1 -- Voltage Measurement2/LConn2
  Voltage Measurement2/LConn1 -- VMeasure/RConn1

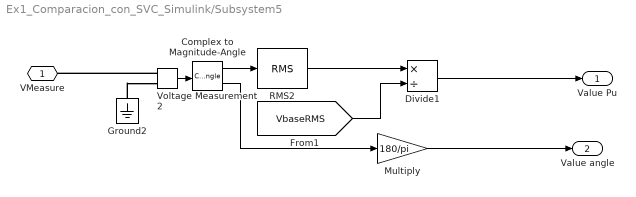
== system Ex1_Comparacion_con_SVC_Simulink/Subsystem5 ==
  Complex to Magnitude-Angle : ComplexToMagnitudeAngle
  Divide1 : Product  Inputs=*/
  Ground2 : powerlib/Elements/Ground  LConnTagsString=a
      settings: SourceProductName=Simscape Electrical
  Multiply : Gain  Gain=180/pi
  RMS2 : powerlib_meascontrol/Measurements/RMS  TrueRMS=on  Freq=60  RMSInit=120  Ts=0
      settings: SourceProductName=Simscape Electrical
  Voltage Measurement2 : powerlib/Measurements/Voltage Measurement  PhasorSimulation=on  OutputType=Complex  PSBequivalent=0
      settings: SourceProductName=Simscape Electrical
  VMeasure : PMIOPort  Side=Left
  "Value Pu " : Outport
  Value angle : Outport  Port=2
  wires:
  RMS2/1 -> Divide1/1
  Divide1/1 -> "Value Pu "/1
  [VbaseRMS] -> Divide1/2
  Voltage Measurement2/1 -> Complex to Magnitude-Angle/1
  Complex to Magnitude-Angle/1 -> RMS2/1
  Multiply/1 -> Value angle/1
  Complex to Magnitude-Angle/2 -> Multiply/1
  connections:
  Ground2/LConn1 -- Voltage Measurement2/LConn2
  Voltage Measurement2/LConn1 -- VMeasure/RConn1

== system Ex1_Comparacion_con_SVC_Simulink/Subsystem6 ==
  Complex to Magnitude-Angle : ComplexToMagnitudeAngle
  Divide1 : Product  Inputs=*/
  Ground2 : powerlib/Elements/Ground  LConnTagsString=a
      settings: SourceProductName=Simscape Electrical
  Multiply : Gain  Gain=180/pi
  RMS2 : powerlib_meascontrol/Measurements/RMS  TrueRMS=on  Freq=60  RMSInit=120  Ts=0
      settings: SourceProductName=Simscape Electrical
  Voltage Measurement2 : powerlib/Measurements/Voltage Measurement  PhasorSimulation=on  OutputType=Complex  PSBequivalent=0
      settings: SourceProductName=Simscape Electrical
  VMeasure : PMIOPort  Side=Left
  "Value Pu " : Outport
  Value angle : Outport  Port=2
  wires:
  RMS2/1 -> Divide1/1
  Divide1/1 -> "Value Pu "/1
  [VbaseRMS] -> Divide1/2
  Voltage Measurement2/1 -> Complex to Magnitude-Angle/1
  Complex to Magnitude-Angle/1 -> RMS2/1
  Multiply/1 -> Value angle/1
  Complex to Magnitude-Angle/2 -> Multiply/1
  connections:
  Ground2/LConn1 -- Voltage Measurement2/LConn2
  Voltage Measurement2/LConn1 -- VMeasure/RConn1
